simulink model "fuzzy_control_car_chasing"  (Simulink 10.1)
settings: Solver=ode3  StartTime=0.0  StopTime=50  FixedStep=0.1  RelTol=1e-3  EnableMultiTasking=on
libraries: simulink_extras x1, fuzblock x1
settings Model: Creator=aa  LastModifiedBy=78253
settings DataIOCC: LimitDataPoints=on  SignalLoggingSaveFormat=ModelDataLogs  SignalLoggingName=sigsOut
settings OptimizationCC: InitFltsAndDblsToZero=on
settings DebuggingCC: SaveWithParameterizedLinksMsg=none  SignalResolutionControl=TryResolveAllWithWarning  MultiTaskDSMMsg=warning  MultiTaskCondExecSysMsg=none  FcnCallInpInsideContextMsg=warning
settings HardwareCC: TargetUnknown=on
settings GRTTargetCC: TargetFcnLib=ansi_tfl_tmw.mat
settings ConfigComp: CovSFcnEnable=off

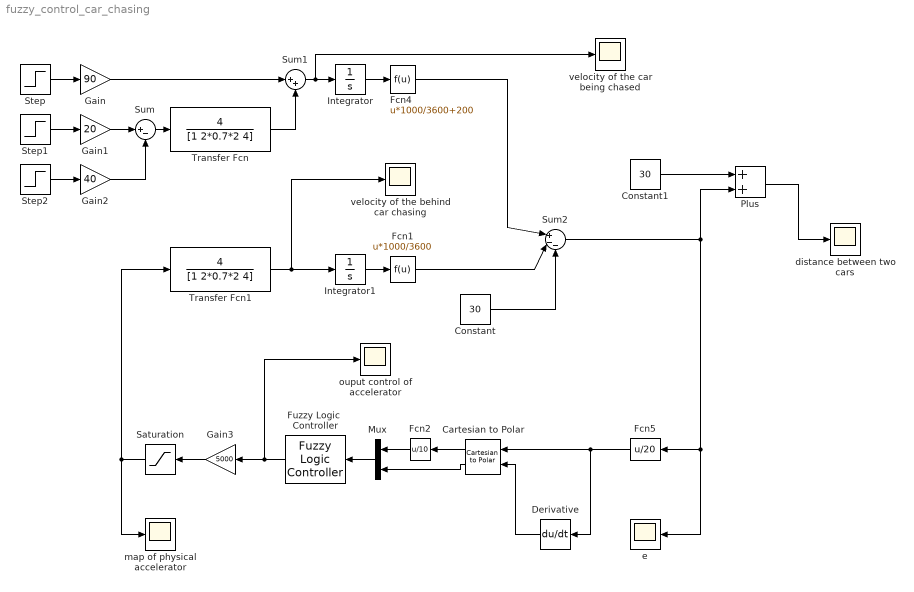
== system fuzzy_control_car_chasing ==
  Cartesian to Polar : simulink_extras/Transformations/Cartesian to Polar
  Constant : Constant  Value=30
  Constant1 : Constant  Value=30
  Derivative : Derivative
  Fcn1 : Fcn  Expr=u*1000/3600
  Fcn2 : Fcn  Expr=u/10
  Fcn4 : Fcn  Expr=u*1000/3600+200
  Fcn5 : Fcn  Expr=u/20
  Fuzzy Logic  Controller : fuzblock/Fuzzy Logic  Controller  FIS='carf5.fis'  OutputSampleNumber=101  DataType=double  FuzzifiedInputs=off  RuleFiringStrengths=off  RuleOutputs=off  AggregatedOutputs=off  SimulateUsing=Interpreted execution  OutOfRangeInputValueMessage=warning  NoRuleFiredMessage=warning  EmptyOutputFuzzySetMessage=warning
  Gain : Gain  Gain=90  SaturateOnIntegerOverflow=on  OutDataTypeStr=Inherit: Same as input  ParamDataTypeStr=Inherit: Same as input
  Gain1 : Gain  Gain=20  SaturateOnIntegerOverflow=on  OutDataTypeStr=Inherit: Same as input  ParamDataTypeStr=Inherit: Same as input
  Gain2 : Gain  Gain=40  SaturateOnIntegerOverflow=on  OutDataTypeStr=Inherit: Same as input  ParamDataTypeStr=Inherit: Same as input
  Gain3 : Gain  Gain=5000  SaturateOnIntegerOverflow=on  OutDataTypeStr=Inherit: Same as input  ParamDataTypeStr=Inherit: Same as input
  Integrator : Integrator
  Integrator1 : Integrator
  Mux : Mux  Inputs=2
  Plus : Sum
  Saturation : Saturate  UpperLimit=200  LowerLimit=0
  Step : Step  Time=0  SampleTime=0
  Step1 : Step  Time=25  SampleTime=0
  Step2 : Step  Time=35  SampleTime=0
  Sum : Sum  Inputs=|+-  SaturateOnIntegerOverflow=on
  Sum1 : Sum  Inputs=|++  SaturateOnIntegerOverflow=on
  Sum2 : Sum  Inputs=|+--  SaturateOnIntegerOverflow=on
  Transfer Fcn : TransferFcn  Numerator=[4]  Denominator=[1 2*0.7*2 4]
  Transfer Fcn1 : TransferFcn  Numerator=[4]  Denominator=[1 2*0.7*2 4]
  distance between two cars : Scope
  e : Scope
  map of physical accelerator : Scope
  ouput control of accelerator : Scope
  velocity of the behind car chasing : Scope
  velocity of the car being chased : Scope
  wires:
  Step/1 -> Gain/1
  Step1/1 -> Gain1/1
  Step2/1 -> Gain2/1
  Sum/1 -> Transfer Fcn/1
  Integrator/1 -> Fcn4/1
  Constant/1 -> Sum2/3
  Sum2/1 -> Fcn5/1, e/1, Plus/2
  Derivative/1 -> Cartesian to Polar/2
  Cartesian to Polar/2 -> Mux/2
  Mux/1 -> Fuzzy Logic  Controller/1
  Fcn1/1 -> Sum2/2
  Fcn4/1 -> Sum2/1
  Integrator1/1 -> Fcn1/1
  Fcn5/1 -> Derivative/1, Cartesian to Polar/1
  Transfer Fcn1/1 -> Integrator1/1, velocity of the behind car chasing/1
  Transfer Fcn/1 -> Sum1/2
  Sum1/1 -> velocity of the car being chased/1, Integrator/1
  Gain/1 -> Sum1/1
  Gain1/1 -> Sum/1
  Gain2/1 -> Sum/2
  Cartesian to Polar/1 -> Fcn2/1
  Fcn2/1 -> Mux/1
  Fuzzy Logic  Controller/1 -> ouput control of accelerator/1, Gain3/1
  Gain3/1 -> Saturation/1
  Saturation/1 -> Transfer Fcn1/1, map of physical accelerator/1
  Constant1/1 -> Plus/1
  Plus/1 -> distance between two cars/1
